simulink model "waterTank1"  (R2015a)
settings: Solver=ode45  StartTime=0.0  StopTime=24*3600*4  RelTol=1e-3
undefined symbols (not defined in the file): A, H
settings Model: Creator=student  LastModifiedBy=student

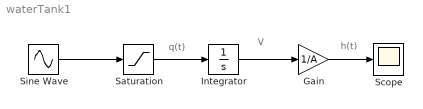
== system waterTank1 ==
  note: q(t)
  note: V
  note: h(t)
  Gain : Gain  Gain=1/A
  Integrator : Integrator  LimitOutput=on  UpperSaturationLimit=A*H  LowerSaturationLimit=0
  Saturation : Saturate  UpperLimit=inf  LowerLimit=0
  Scope : Scope
  Sine Wave : Sin  Amplitude=5/(60*1000)  Frequency=2*pi/(24*3600)  SampleTime=0
  wires:
  Sine Wave/1 -> Saturation/1
  Saturation/1 -> Integrator/1
  Integrator/1 -> Gain/1
  Gain/1 -> Scope/1
